simulink model "model"  (R2019a)
settings: Solver=VariableStepAuto  StartTime=0.0  StopTime=10.0  RelTol=1e-3
values from neighbouring files (symbols this model uses):
  Ixx = I(1)    [setup.m]
  Ixz = I(3)    [setup.m]
  Iyy = I(4)    [setup.m]
  Izz = I(6)    [setup.m]
undefined symbols (not defined in the file or in its folder): sigbuilder_block
settings Model: Creator=rafal  LastModifiedBy=rafal
settings DataIOCC: ReturnWorkspaceOutputs=off
settings DebuggingCC: ArithmeticOperatorsInVariantConditions=warning

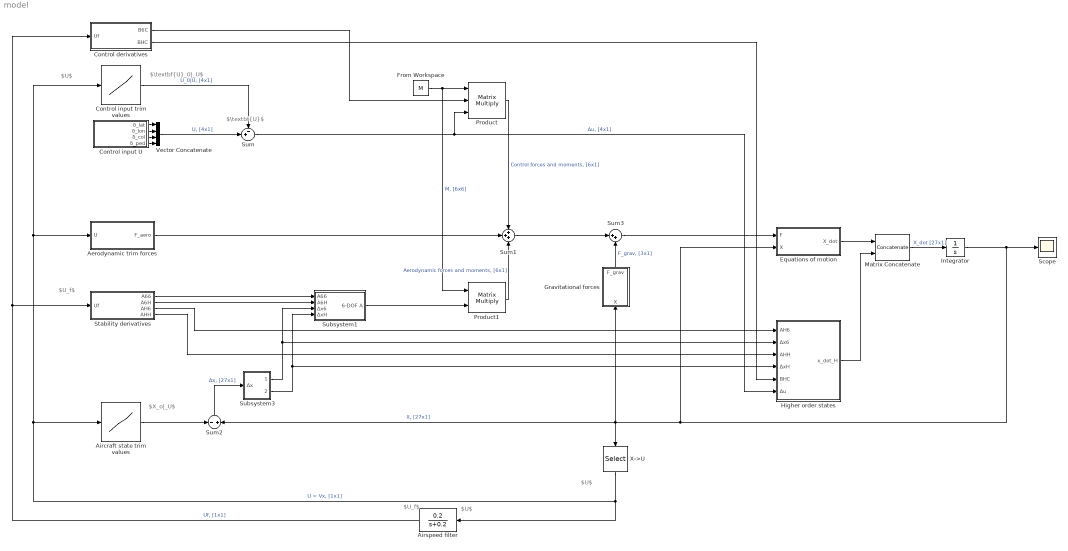
== system model ==
  note: $U$
  note: $U_f$
  note: $X_o|_U$
  note: $U_f$
  note: $U$
  note: $U$
  note: $\textbf{U}$
  note: $\textbf{U}_0|_U$
  Aerodynamic trim forces : Subsystem
  Aircraft state trim values : Lookup_n-D  NumberOfTableDimensions=1  BreakpointsForDimension3=[5, 7]  Table=reshape(repmat([4 5 6;16 19 20;10 18 23],1,2),[3,3,2])  InternalRulePriority=Speed  RndMeth=Simplest  InputSameDT=on
  Airspeed filter : TransferFcn  Numerator=[0.2]  Denominator=[1 0.2]  ContinuousStateAttributes="\""
  Control derivatives : Subsystem
  Control input U : Subsystem  Tag=STV Subsys  LoadFcn=sigbuilder_block('load');  StartFcn=sigbuilder_block('start');  StopFcn=sigbuilder_block('stop');  ClipboardFcn=sigbuilder_block('clipboard');  mask(Sigbuilder block){tuvar=[0:10]}
      mask help: Simulink:masks:SigbuilderBlock_MD
      mask init:
      | if ~strcmp(get_param(bdroot(gcbh),'SimulationStatus'),'stopped') tuvar = sigbuilder_block('maskInit'); end
      settings: CopyFcn=sigbuilder_block('copy');  DeleteFcn=sigbuilder_block('delete');  ModelCloseFcn=sigbuilder_block('modelClose');  PreSaveFcn=sigbuilder_block('preSave');  PauseFcn=sigbuilder_block('pause');  ContinueFcn=sigbuilder_block('continue');  NameChangeFcn=sigbuilder_block('namechange');  OpenFcn=sigbuilder_block('open',[642.75 122.25 550.5 399.75 ]);  CloseFcn=sigbuilder_block('close');
      mask Display: plot(0, 0, 100, 100,[2, 2, 32, 32, 2], [68, 8, 8, 68, 68],[32, 2], [38, 38], [32, 19, 2],[53, 60, 44], [32, 17, 17, 2],[16, 16, 31, 31]);txt = getActiveGroup(gcbh);text(2, 100, txt,'verticalAlignment', 'top');
  Control input trim values : Lookup_n-D  NumberOfTableDimensions=1  BreakpointsForDimension3=[5, 7]  Table=reshape(repmat([4 5 6;16 19 20;10 18 23],1,2),[3,3,2])  InternalRulePriority=Speed  RndMeth=Simplest  InputSameDT=on
  Equations of motion : Subsystem
  From Workspace : FromWorkspace  VariableName=M  SampleTime=0
  Gravitational forces : Subsystem
  Higher order states : Subsystem
  Integrator : Integrator
  Matrix Concatenate : Concatenate  Mode=Multidimensional array
  Product : Product  Inputs=3  Multiplication=Matrix(*)
  Product1 : Product  Multiplication=Matrix(*)
  Scope : Scope
  Stability derivatives : Subsystem
  Subsystem1 : Subsystem
  Subsystem3 : Subsystem
  Sum : Sum  Inputs=-+|
  Sum1 : Sum  Inputs=+++
  Sum2 : Sum  Inputs=-+
  Sum3 : Sum  Inputs=|++
  Vector Concatenate : Concatenate  NumInputs=4  Mode=Multidimensional array
  X->U : Selector  InputPortWidth=9  IndexOptions=Index vector (dialog)  Indices=[1]  OutputSizes=1
  wires:
  Control input trim values/1 -> Sum/1  "U_0|U, [4x1]"
  Control input U/1(δ_lat) -> Vector Concatenate/1
  Vector Concatenate/1 -> Sum/2  "U, [4x1]"
  Control input U/2(δ_lon) -> Vector Concatenate/2
  Control input U/3(δ_col) -> Vector Concatenate/3
  Control input U/4(δ_ped) -> Vector Concatenate/4
  Sum/1 -> Product/3, Higher order states/6(∆u)  "∆u, [4x1]"
  Product/1 -> Sum1/1  "Control forces and moments, [6x1]"
  Product1/1 -> Sum1/3  "Aerodynamic forces and moments, [6x1]"
  Aircraft state trim values/1 -> Sum2/1
  Airspeed filter/1 -> Stability derivatives/1(Uf), Control derivatives/1(Uf)  "Uf, [1x1]"
  Sum1/1 -> Sum3/1
  Sum3/1 -> Equations of motion/1(F)
  Integrator/1 -> Scope/1, Sum2/2, Gravitational forces/1(X), X->U/1, Equations of motion/2(X)  "X, [27x1]"
  X->U/1 -> Aerodynamic trim forces/1(U), Control input trim values/1, Aircraft state trim values/1, Airspeed filter/1  "U = Vx, [1x1]"
  Aerodynamic trim forces/1(F_aero) -> Sum1/2
  Gravitational forces/1(F_grav) -> Sum3/2  "F_grav, [3x1]"
  From Workspace/1 -> Product1/1, Product/1  "M, [6x6]"
  Stability derivatives/1(A66) -> Subsystem1/1(A66)
  Stability derivatives/2(A6H) -> Subsystem1/2(A6H)
  Subsystem1/1(6-DOF A) -> Product1/2
  Control derivatives/1(B6C) -> Product/2
  Stability derivatives/3(AH6) -> Higher order states/1(AH6)
  Sum2/1 -> Subsystem3/1(∆x)  "∆x, [27x1]"
  Subsystem3/1(∆x6) -> Subsystem1/3(∆x6), Higher order states/2(∆x6)
  Subsystem3/2(∆xH) -> Higher order states/4(∆xH), Subsystem1/4(∆xH)
  Stability derivatives/4(AHH) -> Higher order states/3(AHH)
  Control derivatives/2(BHC) -> Higher order states/5(BHC)
  Matrix Concatenate/1 -> Integrator/1  "X_dot [27x1]"
  Equations of motion/1(X_dot) -> Matrix Concatenate/1
  Higher order states/1(x_dot_H) -> Matrix Concatenate/2

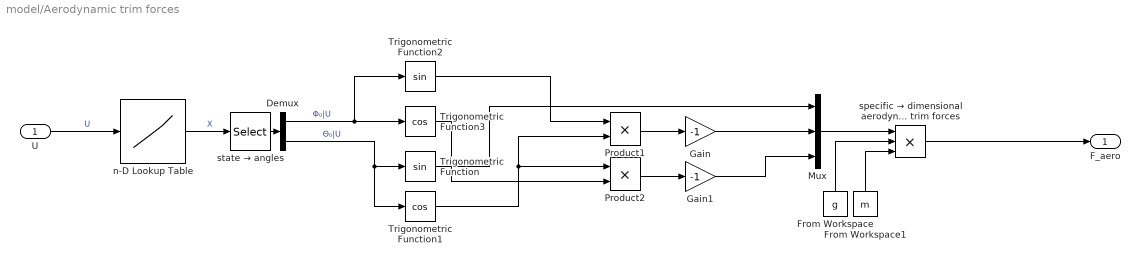
== system model/Aerodynamic trim forces ==
  U : Inport
  Demux : Demux  Outputs=2
  From Workspace : FromWorkspace  VariableName=g  SampleTime=0
  From Workspace1 : FromWorkspace  VariableName=m  SampleTime=0
  Gain : Gain  Gain=-1
  Gain1 : Gain  Gain=-1
  Mux : Mux  Inputs=3
  Product1 : Product
  Product2 : Product
  Trigonometric Function : Trigonometry
  Trigonometric Function1 : Trigonometry  Operator=cos
  Trigonometric Function2 : Trigonometry
  Trigonometric Function3 : Trigonometry  Operator=cos
  n-D Lookup Table : Lookup_n-D  NumberOfTableDimensions=1  BreakpointsForDimension3=[5, 7]  Table=reshape(repmat([4 5 6;16 19 20;10 18 23],1,2),[3,3,2])  InternalRulePriority=Speed  RndMeth=Simplest  InputSameDT=on
  specific → dimensional aerodynamic trim forces : Product  Inputs=3
  state → angles : Selector  InputPortWidth=9  IndexOptions=Index vector (dialog)  Indices=[7 8]  OutputSizes=1
  F_aero : Outport
  wires:
  n-D Lookup Table/1 -> state → angles/1  "X"
  state → angles/1 -> Demux/1
  Demux/1 -> Trigonometric Function2/1, Trigonometric Function3/1  "Φ₀|U"
  Demux/2 -> Trigonometric Function1/1, Trigonometric Function/1  "Θ₀|U"
  Product2/1 -> Gain1/1
  Product1/1 -> Gain/1
  Trigonometric Function1/1 -> Product2/1, Product1/2
  Trigonometric Function2/1 -> Product1/1
  Trigonometric Function3/1 -> Product2/2
  Gain/1 -> Mux/2
  Trigonometric Function/1 -> Mux/1
  Gain1/1 -> Mux/3
  U/1 -> n-D Lookup Table/1  "U"
  Mux/1 -> specific → dimensional aerodynamic trim forces/1
  From Workspace1/1 -> specific → dimensional aerodynamic trim forces/3
  specific → dimensional aerodynamic trim forces/1 -> F_aero/1
  From Workspace/1 -> specific → dimensional aerodynamic trim forces/2

== system model/Control derivatives ==
  Uf : Inport
  Control derivatives lookup : Lookup_n-D  NumberOfTableDimensions=1  BreakpointsForDimension3=[5, 7]  Table=reshape(repmat([4 5 6;16 19 20;10 18 23],1,2),[3,3,2])  InternalRulePriority=Speed  RndMeth=Simplest  InputSameDT=on
  Selector : Selector  NumberOfDimensions=2  InputPortWidth=3  IndexOptions=Starting index (dialog),Starting index (dialog)  Indices=1,1  OutputSizes=6,4
  Selector1 : Selector  NumberOfDimensions=2  InputPortWidth=3  IndexOptions=Starting index (dialog),Starting index (dialog)  Indices=7,1  OutputSizes=21,4
  B6C : Outport
  BHC : Outport  Port=2
  wires:
  Selector1/1 -> BHC/1
  Selector/1 -> B6C/1
  Uf/1 -> Control derivatives lookup/1
  Control derivatives lookup/1 -> Selector1/1, Selector/1

== system model/Control input U ==
  Demux : Demux  Tag=STV Demux
  FromWs : FromWorkspace  Tag=STV FromWs  VariableName=tuvar  SampleTime=0
      SigBuilderData=|
      | common.afterFinalStr = 'Extrapolate'
      | common.sampleTime = 0
      | dataSet.timeRange = [0 10]
      | dataSet.name = 'Group 1'
      | sbobj.Groups.Name = 'Group 1'
      | sbobj.Groups.Signals(1).Name = 'δ_lat'
      | sbobj.Groups.Signals(1).XData = [0 4 4 6 6 10]
      | sbobj.Groups.Signals(1).YData = [-0.005 0.385 1 1 0.635 0.635]
      | sbobj.Groups.Signals(2).Name = 'δ_lon'
      | sbobj.Groups.Signals(2).XData = [0 5 5 10]
      | sbobj.Groups.Signals(2).YData = [0 0 1 1]
      | sbobj.Groups.Signals(3).Name = 'δ_col'
      | sbobj.Groups.Signals(3).XData = [0 2.98 2.98 10]
      | sbobj.Groups.Signals(3).YData = [0 0 1 1]
      | sbobj.Groups.Signals(4).Name = 'δ_ped'
      | sbobj.Groups.Signals(4).XData = [0 4 4 6 6 10]
      | sbobj.Groups.Signals(4).YData = [0 0 1 1 0 0]
  δ_lat : Outport  Tag=STV Outport
  δ_lon : Outport  Tag=STV Outport  Port=2
  δ_col : Outport  Tag=STV Outport  Port=3
  δ_ped : Outport  Tag=STV Outport  Port=4
  wires:
  Demux/1 -> δ_lat/1
  FromWs/1 -> Demux/1
  Demux/2 -> δ_lon/1
  Demux/3 -> δ_col/1
  Demux/4 -> δ_ped/1

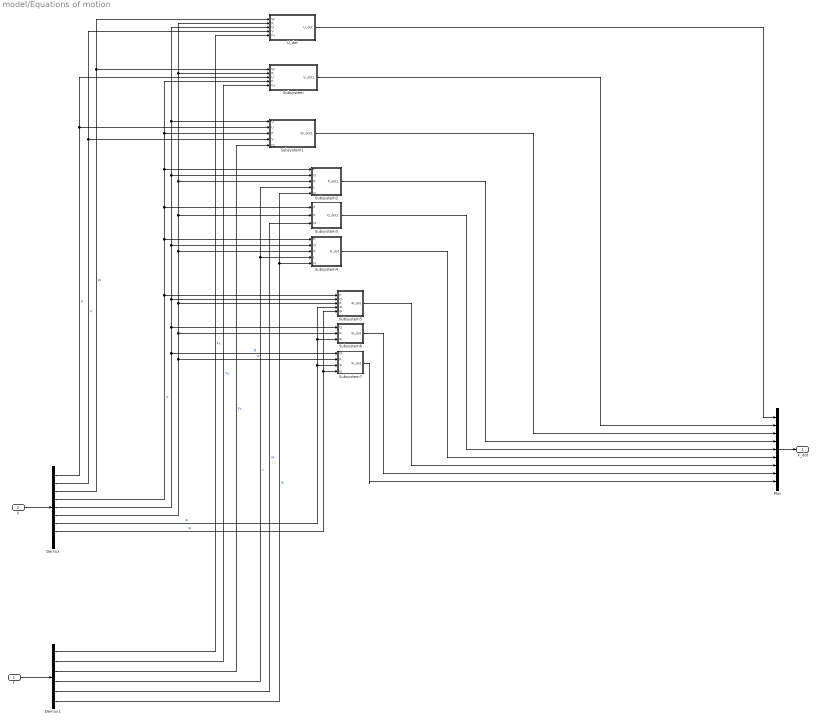
== system model/Equations of motion ==
  F : Inport
  X : Inport  Port=2
  Demux : Demux  Outputs=9
  Demux1 : Demux  Outputs=6
  Mux : Mux  Inputs=9
  Subsystem : Subsystem
  Subsystem1 : Subsystem
  Subsystem2 : Subsystem
  Subsystem3 : Subsystem
  Subsystem4 : Subsystem
  Subsystem5 : Subsystem
  Subsystem6 : Subsystem
  Subsystem7 : Subsystem
  U_dot : Subsystem
  X_dot : Outport
  wires:
  X/1 -> Demux/1
  Demux/1 -> Subsystem/3(U), Subsystem1/2(U)  "U"
  Demux/2 -> U_dot/4(V), Subsystem1/4(V)  "V"
  Demux/3 -> U_dot/1(W), Subsystem/1(W)  "W"
  Demux/4 -> Subsystem/4(P), Subsystem1/3(P), Subsystem2/1(P), Subsystem3/1(P), Subsystem4/1(P), Subsystem5/1(P)  "P"
  Demux/5 -> Subsystem7/1(Q), Subsystem5/2(Q), U_dot/3(Q), Subsystem1/1(Q), Subsystem2/2(Q), Subsystem4/2(Q), Subsystem6/1(Q)  "Q"
  Demux/6 -> Subsystem7/2(R), Subsystem6/2(R), Subsystem5/3(R), U_dot/2(R), Subsystem/2(R), Subsystem2/3(R), Subsystem3/2(R), Subsystem4/3(R)  "R"
  Mux/1 -> X_dot/1
  F/1 -> Demux1/1
  Demux1/1 -> U_dot/5(Fx)  "Fx"
  U_dot/1(U_dot) -> Mux/1
  Demux1/2 -> Subsystem/5(Fy)  "Fy"
  Subsystem/1(V_dot1) -> Mux/2
  Demux1/3 -> Subsystem1/5(Fz)  "Fz"
  Subsystem1/1(W_dot1) -> Mux/3
  Demux1/4 -> Subsystem2/4(L), Subsystem4/4(L)  "L"
  Demux1/6 -> Subsystem2/5(N), Subsystem4/5(N)  "N"
  Subsystem2/1(P_dot1) -> Mux/4
  Demux1/5 -> Subsystem3/3(M)  "M"
  Subsystem3/1(Q_dot1) -> Mux/5
  Subsystem4/1(R_dot) -> Mux/6
  Demux/7 -> Subsystem7/3(Φ), Subsystem6/3(Φ), Subsystem5/4(Φ)  "Φ"
  Demux/8 -> Subsystem7/4(Θ), Subsystem5/5(Θ)  "Θ"
  Subsystem5/1(Φ_dot) -> Mux/7
  Subsystem6/1(Θ_dot) -> Mux/8
  Subsystem7/1(Ψ_dot) -> Mux/9

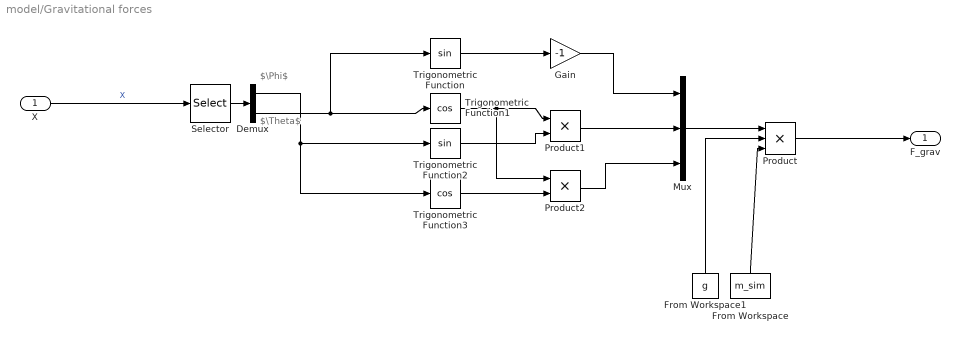
== system model/Gravitational forces ==
  note: $\Phi$
  note: $\Theta$
  X : Inport
  Demux : Demux  Outputs=2
  From Workspace : FromWorkspace  VariableName=m_sim  SampleTime=0
  From Workspace1 : FromWorkspace  VariableName=g  SampleTime=0
  Gain : Gain  Gain=-1
  Mux : Mux  Inputs=3
  Product : Product  Inputs=3
  Product1 : Product
  Product2 : Product
  Selector : Selector  InputPortWidth=9  IndexOptions=Index vector (dialog)  Indices=[7 8]  OutputSizes=1
  Trigonometric Function : Trigonometry
  Trigonometric Function1 : Trigonometry  Operator=cos
  Trigonometric Function2 : Trigonometry
  Trigonometric Function3 : Trigonometry  Operator=cos
  F_grav : Outport
  wires:
  X/1 -> Selector/1  "X"
  Selector/1 -> Demux/1
  Mux/1 -> Product/1
  From Workspace/1 -> Product/3
  From Workspace1/1 -> Product/2
  Demux/2 -> Trigonometric Function/1, Trigonometric Function1/1
  Trigonometric Function/1 -> Gain/1
  Gain/1 -> Mux/1
  Demux/1 -> Trigonometric Function3/1, Trigonometric Function2/1
  Trigonometric Function1/1 -> Product2/1, Product1/1
  Trigonometric Function2/1 -> Product1/2
  Product1/1 -> Mux/2
  Trigonometric Function3/1 -> Product2/2
  Product2/1 -> Mux/3
  Product/1 -> F_grav/1

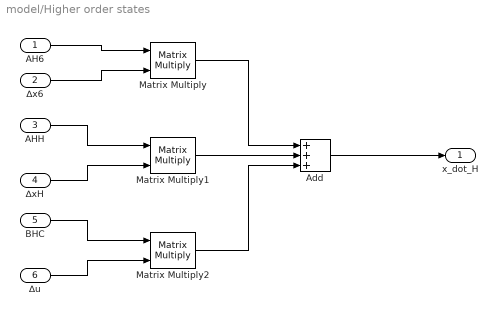
== system model/Higher order states ==
  AH6 : Inport
  ∆x6 : Inport  Port=2
  AHH : Inport  Port=3
  ∆xH : Inport  Port=4
  BHC : Inport  Port=5
  ∆u : Inport  Port=6
  Add : Sum  Inputs=+++
  Matrix Multiply : Product  Multiplication=Matrix(*)
  Matrix Multiply1 : Product  Multiplication=Matrix(*)
  Matrix Multiply2 : Product  Multiplication=Matrix(*)
  x_dot_H : Outport
  wires:
  AH6/1 -> Matrix Multiply/1
  ∆x6/1 -> Matrix Multiply/2
  AHH/1 -> Matrix Multiply1/1
  ∆xH/1 -> Matrix Multiply1/2
  BHC/1 -> Matrix Multiply2/1
  ∆u/1 -> Matrix Multiply2/2
  Matrix Multiply1/1 -> Add/2
  Matrix Multiply/1 -> Add/1
  Matrix Multiply2/1 -> Add/3
  Add/1 -> x_dot_H/1

== system model/Stability derivatives ==
  Uf : Inport
  Selector : Selector  NumberOfDimensions=2  InputPortWidth=3  IndexOptions=Starting index (dialog),Starting index (dialog)  Indices=1,1  OutputSizes=6,6
  Selector1 : Selector  NumberOfDimensions=2  InputPortWidth=3  IndexOptions=Starting index (dialog),Starting index (dialog)  Indices=1,7  OutputSizes=6,21
  Selector2 : Selector  NumberOfDimensions=2  InputPortWidth=3  IndexOptions=Starting index (dialog),Starting index (dialog)  Indices=7,1  OutputSizes=21,6
  Selector3 : Selector  NumberOfDimensions=2  InputPortWidth=3  IndexOptions=Starting index (dialog),Starting index (dialog)  Indices=7,7  OutputSizes=21,21
  Stability derivatives lookup : Lookup_n-D  NumberOfTableDimensions=1  BreakpointsForDimension3=[5, 7]  Table=reshape(repmat([4 5 6;16 19 20;10 18 23],1,2),[3,3,2])  InternalRulePriority=Speed  RndMeth=Simplest  InputSameDT=on
  A66 : Outport
  A6H : Outport  Port=2
  AH6 : Outport  Port=3
  AHH : Outport  Port=4
  wires:
  Selector/1 -> A66/1
  Selector3/1 -> AHH/1
  Selector2/1 -> AH6/1
  Selector1/1 -> A6H/1
  Uf/1 -> Stability derivatives lookup/1
  Stability derivatives lookup/1 -> Selector2/1, Selector3/1, Selector1/1, Selector/1  "A, [27x27]"

== system model/Subsystem1 ==
  A66 : Inport
  A6H : Inport  Port=2
  ∆x6 : Inport  Port=3
  ∆xH : Inport  Port=4
  Add : Sum
  Matrix Multiply : Product  Multiplication=Matrix(*)
  Matrix Multiply1 : Product  Multiplication=Matrix(*)
  6-DOF A : Outport
  wires:
  A66/1 -> Matrix Multiply/1
  A6H/1 -> Matrix Multiply1/1
  Matrix Multiply/1 -> Add/1
  Matrix Multiply1/1 -> Add/2
  Add/1 -> 6-DOF A/1
  ∆x6/1 -> Matrix Multiply/2
  ∆xH/1 -> Matrix Multiply1/2

== system model/Subsystem3 ==
  ∆x : Inport
  Reshape : Reshape  OutputDimensionality=Column vector (2-D)
  Reshape1 : Reshape  OutputDimensionality=Column vector (2-D)
  "∆x6, [6x1]" : Selector  InputPortWidth=27  IndexOptions=Starting index (dialog)  Indices=1  OutputSizes=6
  "∆xH, [21x1]" : Selector  InputPortWidth=27  IndexOptions=Starting index (dialog)  Indices=7  OutputSizes=21
  ∆x6 : Outport
  ∆xH : Outport  Port=2
  wires:
  ∆x/1 -> "∆x6, [6x1]"/1, "∆xH, [21x1]"/1
  "∆x6, [6x1]"/1 -> Reshape/1
  "∆xH, [21x1]"/1 -> Reshape1/1
  Reshape1/1 -> ∆xH/1
  Reshape/1 -> ∆x6/1

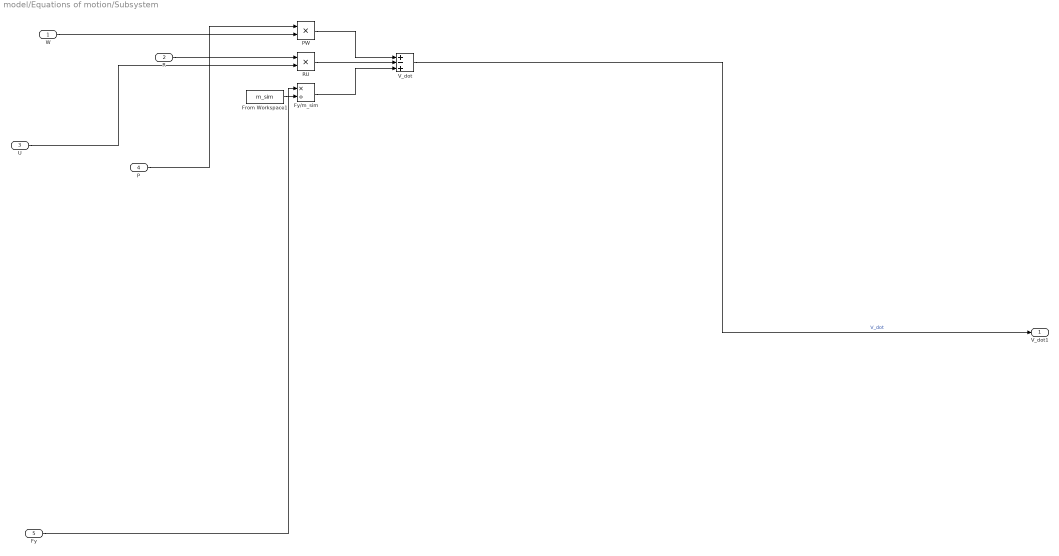
== system model/Equations of motion/Subsystem ==
  W : Inport
  R : Inport  Port=2
  U : Inport  Port=3
  P : Inport  Port=4
  Fy : Inport  Port=5
  From Workspace1 : FromWorkspace  VariableName=m_sim  SampleTime=0
  Fy/m_sim : Product  Inputs=*/
  PW : Product  Inputs=**
  RU : Product  Inputs=**
  V_dot : Sum  Inputs=+-+
  V_dot1 : Outport
  wires:
  Fy/m_sim/1 -> V_dot/3
  V_dot/1 -> V_dot1/1  "V_dot"
  Fy/1 -> Fy/m_sim/1
  PW/1 -> V_dot/1
  P/1 -> PW/1
  U/1 -> RU/2
  RU/1 -> V_dot/2
  From Workspace1/1 -> Fy/m_sim/2
  W/1 -> PW/2
  R/1 -> RU/1

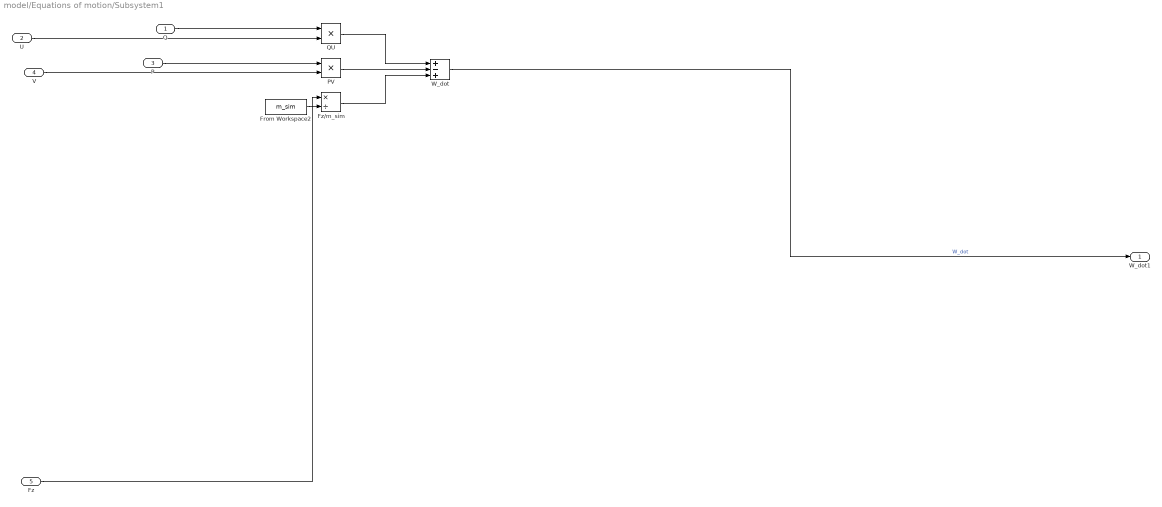
== system model/Equations of motion/Subsystem1 ==
  Q : Inport
  U : Inport  Port=2
  P : Inport  Port=3
  V : Inport  Port=4
  Fz : Inport  Port=5
  From Workspace2 : FromWorkspace  VariableName=m_sim  SampleTime=0
  Fz/m_sim : Product  Inputs=*/
  PV : Product  Inputs=**
  QU : Product  Inputs=**
  W_dot : Sum  Inputs=+-+
  W_dot1 : Outport
  wires:
  Fz/m_sim/1 -> W_dot/3
  U/1 -> QU/2
  V/1 -> PV/2
  QU/1 -> W_dot/1
  Q/1 -> QU/1
  PV/1 -> W_dot/2
  Fz/1 -> Fz/m_sim/1
  From Workspace2/1 -> Fz/m_sim/2
  P/1 -> PV/1
  W_dot/1 -> W_dot1/1  "W_dot"

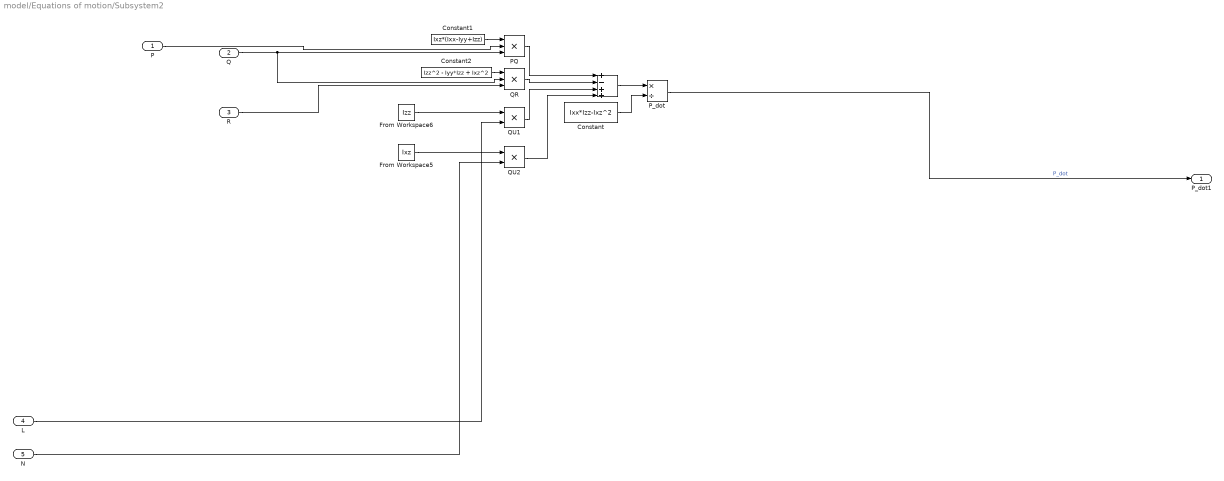
== system model/Equations of motion/Subsystem2 ==
  P : Inport
  Q : Inport  Port=2
  R : Inport  Port=3
  L : Inport  Port=4
  N : Inport  Port=5
  " " : Sum  Inputs=+-++
  Constant : Constant  Value=Ixx*Izz-Ixz^2
  Constant1 : Constant  Value=Ixz*(Ixx-Iyy+Izz)
  Constant2 : Constant  Value=Izz^2 - Iyy*Izz + Ixz^2
  From Workspace5 : FromWorkspace  VariableName=Ixz  SampleTime=0
  From Workspace6 : FromWorkspace  VariableName=Izz  SampleTime=0
  PQ : Product  Inputs=***
  P_dot : Product  Inputs=*/
  QR : Product  Inputs=***
  QU1 : Product  Inputs=**
  QU2 : Product  Inputs=**
  P_dot1 : Outport
  wires:
  From Workspace5/1 -> QU2/1
  P/1 -> PQ/2
  Constant2/1 -> QR/1
  QU1/1 -> " "/3
  PQ/1 -> " "/1
  Constant1/1 -> PQ/1
  " "/1 -> P_dot/1
  QR/1 -> " "/2
  From Workspace6/1 -> QU1/1
  QU2/1 -> " "/4
  Constant/1 -> P_dot/2
  N/1 -> QU2/2
  P_dot/1 -> P_dot1/1  "P_dot"
  L/1 -> QU1/2
  Q/1 -> PQ/3, QR/2
  R/1 -> QR/3

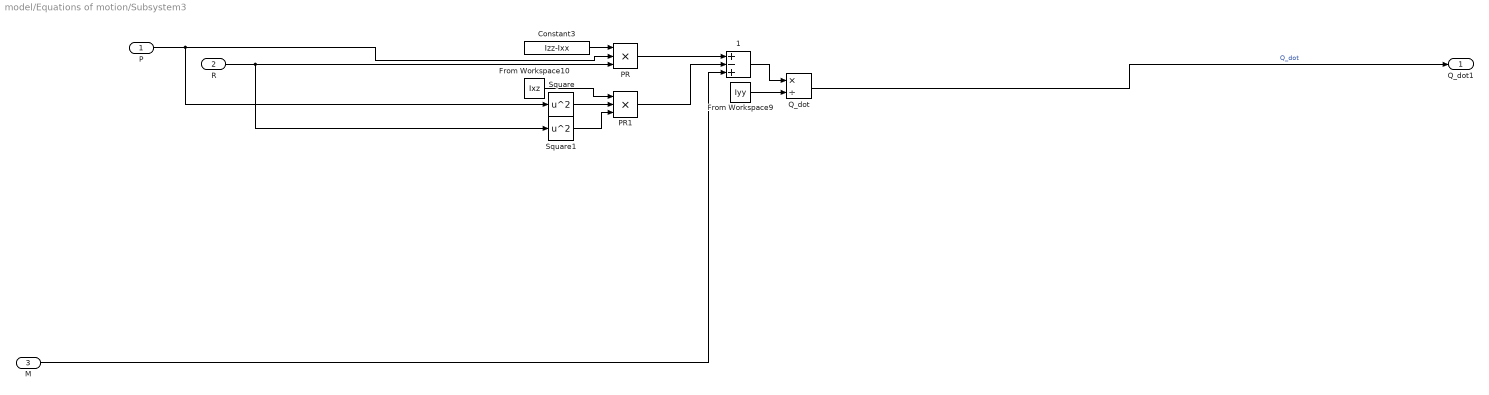
== system model/Equations of motion/Subsystem3 ==
  P : Inport
  R : Inport  Port=2
  M : Inport  Port=3
  " 1" : Sum  Inputs=+-+
  Constant3 : Constant  Value=Izz-Ixx
  From Workspace10 : FromWorkspace  VariableName=Ixz  SampleTime=0
  From Workspace9 : FromWorkspace  VariableName=Iyy  SampleTime=0
  PR : Product  Inputs=***
  PR1 : Product  Inputs=***
  Q_dot : Product  Inputs=*/
  Square : Math  Operator=square  SaturateOnIntegerOverflow=on
  Square1 : Math  Operator=square  SaturateOnIntegerOverflow=on
  Q_dot1 : Outport
  wires:
  From Workspace10/1 -> PR1/1
  From Workspace9/1 -> Q_dot/2
  Square1/1 -> PR1/3
  " 1"/1 -> Q_dot/1
  PR/1 -> " 1"/1
  PR1/1 -> " 1"/2
  R/1 -> Square1/1, PR/3
  Square/1 -> PR1/2
  Constant3/1 -> PR/1
  P/1 -> PR/2, Square/1
  Q_dot/1 -> Q_dot1/1  "Q_dot"
  M/1 -> " 1"/3

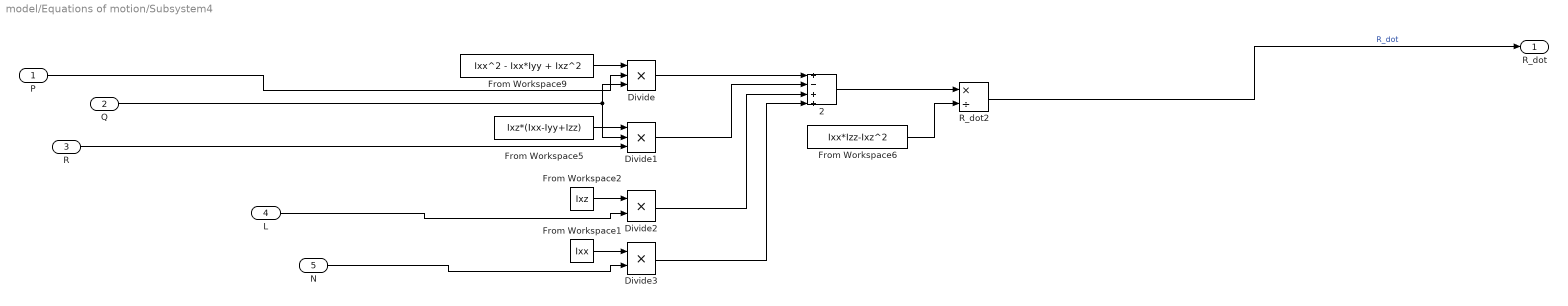
== system model/Equations of motion/Subsystem4 ==
  P : Inport
  Q : Inport  Port=2
  R : Inport  Port=3
  L : Inport  Port=4
  N : Inport  Port=5
  " 2" : Sum  Inputs=+-++
  Divide : Product  Inputs=***
  Divide1 : Product  Inputs=***
  Divide2 : Product  Inputs=**
  Divide3 : Product  Inputs=**
  From Workspace1 : FromWorkspace  VariableName=Ixx  SampleTime=0
  From Workspace2 : FromWorkspace  VariableName=Ixz  SampleTime=0
  From Workspace5 : FromWorkspace  VariableName=Ixz*(Ixx-Iyy+Izz)  SampleTime=0
  From Workspace6 : FromWorkspace  VariableName=Ixx*Izz-Ixz^2  SampleTime=0
  From Workspace9 : FromWorkspace  VariableName=Ixx^2 - Ixx*Iyy + Ixz^2  SampleTime=0
  R_dot2 : Product  Inputs=*/
  R_dot : Outport
  wires:
  Divide/1 -> " 2"/1
  Divide2/1 -> " 2"/3
  Divide1/1 -> " 2"/2
  From Workspace2/1 -> Divide2/1
  Q/1 -> Divide/3, Divide1/2
  From Workspace6/1 -> R_dot2/2
  " 2"/1 -> R_dot2/1
  From Workspace5/1 -> Divide1/1
  From Workspace9/1 -> Divide/1
  L/1 -> Divide2/2
  From Workspace1/1 -> Divide3/1
  Divide3/1 -> " 2"/4
  R/1 -> Divide1/3
  R_dot2/1 -> R_dot/1  "R_dot"
  N/1 -> Divide3/2
  P/1 -> Divide/2

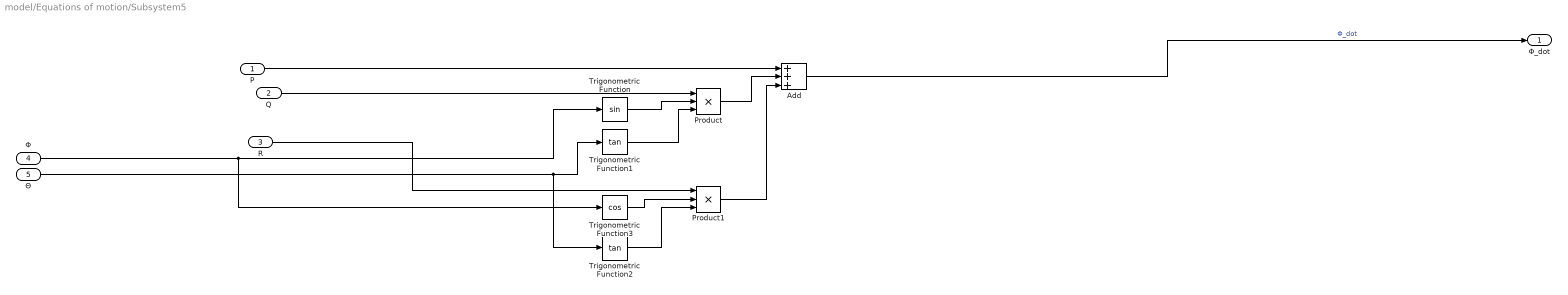
== system model/Equations of motion/Subsystem5 ==
  P : Inport
  Q : Inport  Port=2
  R : Inport  Port=3
  Φ : Inport  Port=4
  Θ : Inport  Port=5
  Add : Sum  Inputs=+++
  Product : Product  Inputs=3
  Product1 : Product  Inputs=3
  Trigonometric Function : Trigonometry
  Trigonometric Function1 : Trigonometry  Operator=tan
  Trigonometric Function2 : Trigonometry  Operator=tan
  Trigonometric Function3 : Trigonometry  Operator=cos
  Φ_dot : Outport
  wires:
  Φ/1 -> Trigonometric Function3/1, Trigonometric Function/1
  Θ/1 -> Trigonometric Function2/1, Trigonometric Function1/1
  Trigonometric Function3/1 -> Product1/2
  P/1 -> Add/1
  Product1/1 -> Add/3
  Add/1 -> Φ_dot/1  "Φ_dot"
  Product/1 -> Add/2
  Trigonometric Function1/1 -> Product/3
  Trigonometric Function2/1 -> Product1/3
  Trigonometric Function/1 -> Product/2
  Q/1 -> Product/1
  R/1 -> Product1/1

== system model/Equations of motion/Subsystem6 ==
  Q : Inport
  R : Inport  Port=2
  Φ : Inport  Port=3
  Product : Product
  Product1 : Product
  Subtract : Sum  Inputs=+-
  Trigonometric Function : Trigonometry  Operator=cos
  Trigonometric Function1 : Trigonometry
  Θ_dot : Outport
  wires:
  R/1 -> Product1/1
  Trigonometric Function/1 -> Product/2
  Φ/1 -> Trigonometric Function1/1, Trigonometric Function/1
  Trigonometric Function1/1 -> Product1/2
  Product/1 -> Subtract/1
  Product1/1 -> Subtract/2
  Q/1 -> Product/1
  Subtract/1 -> Θ_dot/1  "Θ_dot"

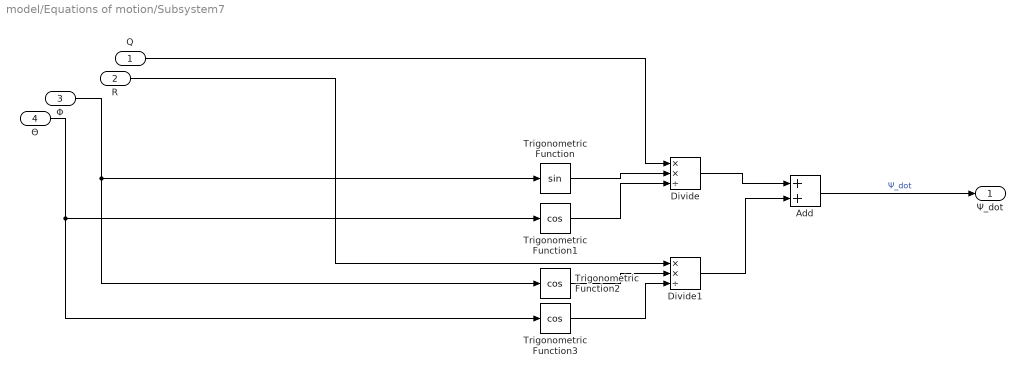
== system model/Equations of motion/Subsystem7 ==
  Q : Inport
  R : Inport  Port=2
  Φ : Inport  Port=3
  Θ : Inport  Port=4
  Add : Sum
  Divide : Product  Inputs=**/
  Divide1 : Product  Inputs=**/
  Trigonometric Function : Trigonometry
  Trigonometric Function1 : Trigonometry  Operator=cos
  Trigonometric Function2 : Trigonometry  Operator=cos
  Trigonometric Function3 : Trigonometry  Operator=cos
  Ψ_dot : Outport
  wires:
  R/1 -> Divide1/1
  Θ/1 -> Trigonometric Function3/1, Trigonometric Function1/1
  Trigonometric Function3/1 -> Divide1/3
  Add/1 -> Ψ_dot/1  "Ψ_dot"
  Φ/1 -> Trigonometric Function2/1, Trigonometric Function/1
  Trigonometric Function2/1 -> Divide1/2
  Divide1/1 -> Add/2
  Trigonometric Function1/1 -> Divide/3
  Trigonometric Function/1 -> Divide/2
  Divide/1 -> Add/1
  Q/1 -> Divide/1

== system model/Equations of motion/U_dot ==
  W : Inport
  R : Inport  Port=2
  Q : Inport  Port=3
  V : Inport  Port=4
  Fx : Inport  Port=5
  From Workspace : FromWorkspace  VariableName=m_sim  SampleTime=0
  Fx/m_sim : Product  Inputs=*/
  QW : Product  Inputs=**
  RV : Product  Inputs=**
  U_dot2 : Sum  Inputs=+-+
  U_dot : Outport
  wires:
  U_dot2/1 -> U_dot/1  "U_dot"
  R/1 -> RV/2
  W/1 -> QW/1
  From Workspace/1 -> Fx/m_sim/2
  QW/1 -> U_dot2/2
  RV/1 -> U_dot2/1
  V/1 -> RV/1
  Fx/m_sim/1 -> U_dot2/3
  Q/1 -> QW/2
  Fx/1 -> Fx/m_sim/1
